simulink model "Position_MPC_Adaptive_OuterLoop"  (R2018a)
settings: Solver=VariableStepAuto  StartTime=0.0  StopTime=inf  FixedStep=0.01  RelTol=1e-3  EnableMultiTasking=on
PreLoadFcn:
  | sampleTime = 0.05;
  | 
  | % Vehicle Parameters
  | R = 0.1;
  | L = 0.5;
undefined symbols (not defined in the file): Ad, Bd, Beta, C1, C2, cBW, d, dw, Kb, Kg, Kt, La, mc, Ra, Waypoint
libraries: mobileRoboticsLib x2, mpclib x1, cstblocks x1, dspsrcs4 x1
settings Model: SimulationMode=accelerator  EnablePacing=on  Creator=scastro  LastModifiedBy=shravan
settings DataIOCC: LimitDataPoints=on
settings OptimizationCC: LifeSpan=inf
settings DebuggingCC: AllowSymbolicDim=off  SFUnexpectedBacktrackingDiag=warning  SFNoUnconditionalDefaultTransitionDiag=warning  SFExecutionAtInitializationDiag=none
settings CodeAppCC: StateflowObjectComments=on
settings GRTTargetCC: TargetLangStandard=C89/C90 (ANSI)  GeneratePreprocessorConditionals=Disable all
settings ConfigComp: CovMetricSettings=dw  CovHtmlReporting=on  CovSaveCumulativeToWorkspaceVar=on  CovSaveSingleToWorkspaceVar=on  CovExternalEMLEnable=off  CovSFcnEnable=off
settings SimscapeCC: SimscapeNominalValues="[{\"value\":\"10\",\"unit\":\"V\"},{\"value\":\"1\",\"unit\":\"A\"},{\"value\":\"10\",\"unit\":\"N*m\"},{\"value\":\"10\",\"unit\":\"bar\"},{\"value\":\"100\",\"unit\":\"kJ/kg\"},{\"value\":\"1\",\"unit\":\"kW\"},{\"value\":\"300\",\"unit\":\"K\"},{\"value\":\"100\",\"unit\":\"cm^3/s\"},{\"value\":\"1\",\"unit\":\"kN\"},{\"value\":\"1\",\"unit\":\"g/cm^3\"},{\"value\":\"1\",\"unit\":\"l\"},{\"value\":\"1\",\"unit\":\"cm^2\"},{\"value\":\"60\",\"unit\":\"Hz\"}]"  SimscapeLogType=all  SimscapeLogDataHistory=10000
settings ConfigurationSet: Description=SimMechanics 2G
settings ExplorerConfigSet: InternalSimMechanicsExplorerSettings="<ExplorerConfiguration><canonicalview>default</canonicalview><AnimationSetting><BasePlaybackSpeed>1.0</BasePlaybackSpeed><PlaybackSpeedFactor>1.0</PlaybackSpeedFactor></AnimationSetting><TilePanel><TileInfo><Tiles Columns=\"1\" Count=\"1\" Rows=\"1\"><Column Weight=\"1\"/><Row Weight=\"1\"/><Tile Height=\"1\" Width=\"1\" X=\"0\" Y=\"0\"/></Tiles></TileInfo><SceneInfo><SceneViewer><BGColor><R>0.60000002384185791</R><G>0.60000002384185791</G><B>0.60000002384185791</B></BGColor><Camera><DoPerspective>off</DoPerspective><Position><X>-1.70656042355848525</X><Y>-0.974920623359631922</Y><Z>4.72930454537082046</Z></Position><Center><X>0.552860638431633689</X><Y>1.42025063411503494</Y><Z>1.4843509506914252</Z></Center><Up><X>0.664249622453917166</X><Y>0.300615402055903091</Y><Z>0.684399604848363485</Z></Up><ViewLimDist>1</ViewLimDist><YLim>2.77881717169207398</YLim><XLim>3.55928742670435394</XLim></Camera></SceneViewer></SceneInfo></TilePanel><MechEditorPanel><Cameras/><GfxPanelCameraMap/><VideoCreator><PlaybackSpeedRatio>1.0</PlaybackSpeedRatio><FrameRate>30</FrameRate><VideoFormat>Motion JPEG AVI</VideoFormat><FrameSize>auto</FrameSize></VideoCreator></MechEditorPanel></ExplorerConfiguration>"

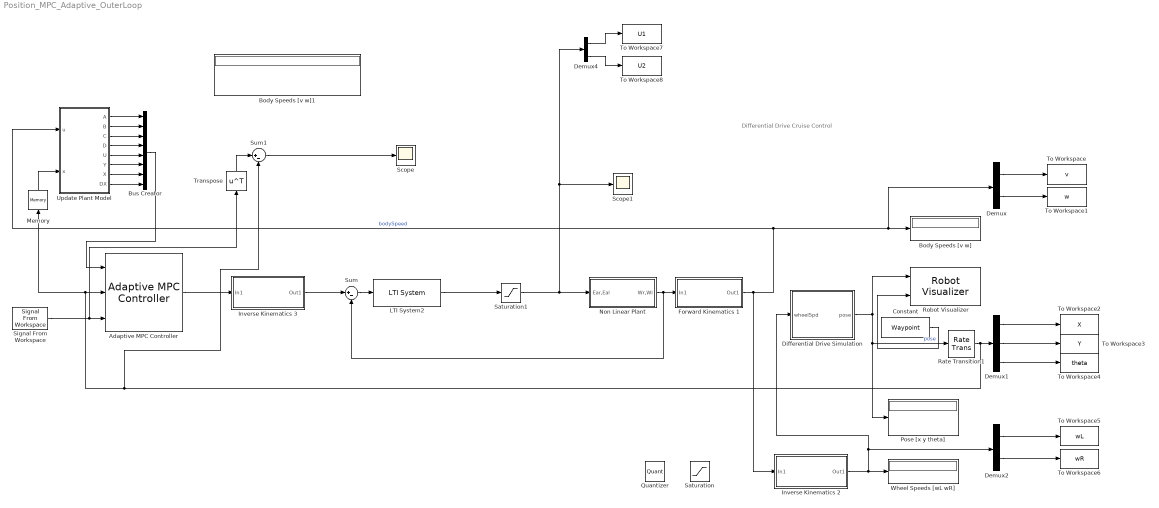
== system Position_MPC_Adaptive_OuterLoop ==
  note: Differential Drive Cruise Control
  Adaptive MPC Controller : mpclib/Adaptive MPC Controller  SCDEnableBlockLinearizationSpecification=on  mpcobj=mpc1  updateMPCinCallerWorkspace=on  md_inport=off  mv_inport=off  cost_outport=off  return_sequence=off  return_qpstatus=off  return_state=off  state_inport=off  isltv_plant=off  lims_inport=off  cc_inport=off  ywt_inport=off  uwt_inport=off  duwt_inport=off  rhoeps_inport=off  uref_inport=off  BlockDataType=double  SampleTimeInherited=off  switch_inport=off
      settings: SourceProductName=Model Predictive Control Toolbox
  Body Speeds [v w] : Display
  Body Speeds [v w]1 : Display
  Bus Creator : BusCreator  Inputs=8
  Constant : Constant  Value=Waypoint  SampleTime=sampleTime
  Demux : Demux  Outputs=2
  Demux1 : Demux  Outputs=3
  Demux2 : Demux  Outputs=2
  Demux4 : Demux  Outputs=2
  Differential Drive Simulation : Subsystem  AncestorBlock=mobileRoboticsLib/Kinematic Models/Differential Drive/Differential Drive Simulation  OverrideUsingVariant=mode==2  mask(Differential Drive Simulation){wheelRadius=R, wheelBase=dw, initX=C1, initY=C2, initAngle=0, Ts=0}
      mask prompts: wheelRadius "Wheel Radius [m]"; wheelBase "Wheelbase [m]"; initX "Initial X Position [m]"; initY "Initial Y Position [m]"; initAngle "Initial Angle [rad]"; Ts "Sample Time"
      mask help:
      | Simulates the kinematics of a differential drive vehicle from a specified initial pose.
      |
      | Input: Left and right wheel speeds [wL; wR], in rad/s
      |
      | Output: Pose [x; y; theta], in m, m, and rad
      |
      | Set the Sample Time parameter to 0 for continuous-time simulation, or a positive number for discrete-time simulation.
      mask Help: web('matlab:edit mrsDocDifferentialDrive')
      mask Callback Ts:
      | Ts = evalin('base',get_param(gcb,'Ts'));
      | blk = [gcb '/Generic Robot Simulation/Velocity Integrator'];
      | if Ts > 0
      |     set_param(blk,'OverrideUsingVariant','mode==2');
      | else
      |     set_param(blk,'OverrideUsingVariant','mode==1');
      | end
  Forward Kinematics 1 : Subsystem
  Inverse Kinematics 2 : Subsystem
  Inverse Kinematics 3 : Subsystem
  LTI System2 : cstblocks/LTI System  sys=Controller  IC=[]
  Memory : Memory
  "Non Linear Plant " : Subsystem
  Pose [x y theta] : Display
  Quantizer : Quantizer
  Rate Transition1 : RateTransition  OutPortSampleTime=0.01
  Robot Visualizer : mobileRoboticsLib/Environments/Robot Visualizer  Priority=99  robotRadius=1  showTrajectory=on  hasWaypoints=on  hasLidar=off  sensorOffset=[ 0 0 ]  scanAngles=[-pi/4,0,pi/4]  hasObjDetector=off  objDetectorOffset=[ 0, 0 ]  objDetectorAngle=0  objDetectorFOV=pi/4  objDetectorMaxRange=5  objectColors=[ 1, 0, 0; 0, 1, 0; 0, 0, 1 ]  objectMarkers='s'
      settings: SourceProductName=Mobile Robotics Simulation Library
  Saturation : Saturate
  Saturation1 : Saturate  UpperLimit=30  LowerLimit=-30
  Scope : Scope
  Scope1 : Scope
  Signal From Workspace : dspsrcs4/Signal From Workspace  X=Lyapunov  Ts=cBW  nsamps=1  OutputAfterFinalValue=Holding final value  ignoreOrWarnInputAndFrameLengths=off  OutputFrames=off
  Sum : Sum  Inputs=|+-
  Sum1 : Sum  Inputs=|+-
  To Workspace : ToWorkspace  VariableName=v  SampleTime=-1
  To Workspace1 : ToWorkspace  VariableName=w  SampleTime=-1
  To Workspace2 : ToWorkspace  VariableName=X  SampleTime=-1
  To Workspace3 : ToWorkspace  VariableName=Y  SampleTime=-1
  To Workspace4 : ToWorkspace  VariableName=theta  SampleTime=-1
  To Workspace5 : ToWorkspace  VariableName=wL  SampleTime=-1
  To Workspace6 : ToWorkspace  VariableName=wR  SampleTime=-1
  To Workspace7 : ToWorkspace  VariableName=U1  SaveFormat=Timeseries  SampleTime=-1
  To Workspace8 : ToWorkspace  VariableName=U2  SaveFormat=Timeseries  SampleTime=-1
  Transpose : Math  Operator=transpose  SaturateOnIntegerOverflow=on
  Update Plant Model : MATLAB Function  TreatAsAtomicUnit=on  SystemSampleTime=0.01
  Wheel Speeds [wL wR] : Display
  wires:
  Differential Drive Simulation/1(pose) -> Rate Transition1/1, Pose [x y theta]/1, Robot Visualizer/1  "pose"
  Forward Kinematics 1/1(Out1) -> Update Plant Model/1(u), Demux/1, Body Speeds [v w]/1, Inverse Kinematics 2/1(In1)  "bodySpeed"
  Demux/1 -> To Workspace/1
  Demux/2 -> To Workspace1/1
  Demux1/1 -> To Workspace2/1
  Demux1/2 -> To Workspace3/1
  Demux2/1 -> To Workspace5/1
  Demux2/2 -> To Workspace6/1
  Constant/1 -> Robot Visualizer/2
  Sum/1 -> LTI System2/1
  Demux1/3 -> To Workspace4/1
  Inverse Kinematics 2/1(Out1) -> Differential Drive Simulation/1(wheelSpd), Demux2/1, Wheel Speeds [wL wR]/1
  "Non Linear Plant "/1(Wr,Wl) -> Forward Kinematics 1/1(In1), Sum/2
  Rate Transition1/1 -> Sum1/2, Memory/1, Adaptive MPC Controller/2, Demux1/1
  Saturation1/1 -> "Non Linear Plant "/1(Ear,Eal), Scope1/1, Demux4/1
  Demux4/1 -> To Workspace7/1
  Demux4/2 -> To Workspace8/1
  Inverse Kinematics 3/1(Out1) -> Sum/1
  LTI System2/1 -> Saturation1/1
  Update Plant Model/1(A) -> Bus Creator/1
  Update Plant Model/2(B) -> Bus Creator/2
  Update Plant Model/3(C) -> Bus Creator/3
  Update Plant Model/4(D) -> Bus Creator/4
  Update Plant Model/5(U) -> Bus Creator/5
  Update Plant Model/6(Y) -> Bus Creator/6
  Update Plant Model/7(X) -> Bus Creator/7
  Update Plant Model/8(DX) -> Bus Creator/8
  Bus Creator/1 -> Adaptive MPC Controller/1
  Memory/1 -> Update Plant Model/2(x)
  Sum1/1 -> Scope/1
  Signal From Workspace/1 -> Transpose/1, Adaptive MPC Controller/3
  Transpose/1 -> Sum1/1
  Adaptive MPC Controller/1 -> Inverse Kinematics 3/1(In1)

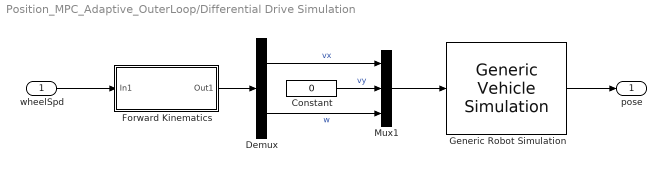
== system Position_MPC_Adaptive_OuterLoop/Differential Drive Simulation ==
  wheelSpd : Inport
  Constant : Constant  Value=0
  Demux : Demux  Outputs=2
  "Forward Kinematics " : Subsystem
  Generic Robot Simulation : mobileRoboticsLib/Utilities/Generic Vehicle Simulation  initX=initX  initY=initY  initAngle=initAngle  Ts=Ts
      link override Velocity Integrator: OverrideUsingVariant=mode==1
      settings: SourceProductName=Mobile Robotics Simulation Toolbox
  Mux1 : Mux  Inputs=3
  pose : Outport
  wires:
  Generic Robot Simulation/1 -> pose/1
  "Forward Kinematics "/1(Out1) -> Demux/1
  wheelSpd/1 -> "Forward Kinematics "/1(In1)
  Constant/1 -> Mux1/2  "vy"
  Demux/2 -> Mux1/3  "w"
  Demux/1 -> Mux1/1  "vx"
  Mux1/1 -> Generic Robot Simulation/1

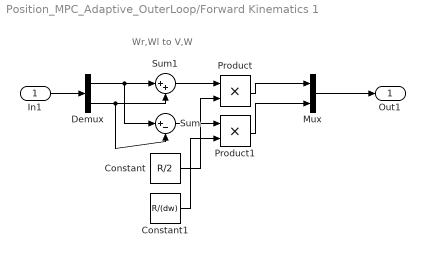
== system Position_MPC_Adaptive_OuterLoop/Forward Kinematics 1 ==
  note: Wr,Wl to V,W
  In1 : Inport
  Constant : Constant  Value=R/2
  Constant1 : Constant  Value=R/(dw)
  Demux : Demux  Outputs=2
  Mux : Mux  Inputs=2
  Product : Product
  Product1 : Product
  Sum : Sum  Inputs=|+-
  Sum1 : Sum  Inputs=|++
  Out1 : Outport
  wires:
  Constant1/1 -> Product1/2
  Sum/1 -> Product1/1
  Constant/1 -> Product/2
  Sum1/1 -> Product/1
  Demux/2 -> Sum1/2, Sum/2
  Demux/1 -> Sum1/1, Sum/1
  Product/1 -> Mux/1
  Mux/1 -> Out1/1
  Product1/1 -> Mux/2
  In1/1 -> Demux/1

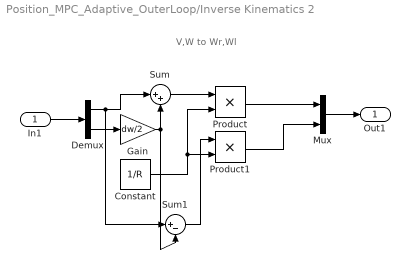
== system Position_MPC_Adaptive_OuterLoop/Inverse Kinematics 2 ==
  note: V,W to Wr,Wl
  In1 : Inport
  Constant : Constant  Value=1/R
  Demux : Demux  Outputs=2
  Gain : Gain  Gain=dw/2
  Mux : Mux  Inputs=2
  Product : Product
  Product1 : Product
  Sum : Sum  Inputs=|++
  Sum1 : Sum  Inputs=|+-
  Out1 : Outport
  wires:
  Gain/1 -> Sum/2, Sum1/2
  Product1/1 -> Mux/2
  Product/1 -> Mux/1
  Sum1/1 -> Product1/1
  Constant/1 -> Product/2, Product1/2
  Sum/1 -> Product/1
  Demux/1 -> Sum/1, Sum1/1
  Demux/2 -> Gain/1
  In1/1 -> Demux/1
  Mux/1 -> Out1/1

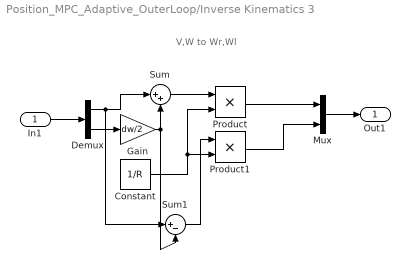
== system Position_MPC_Adaptive_OuterLoop/Inverse Kinematics 3 ==
  note: V,W to Wr,Wl
  In1 : Inport
  Constant : Constant  Value=1/R
  Demux : Demux  Outputs=2
  Gain : Gain  Gain=dw/2
  Mux : Mux  Inputs=2
  Product : Product
  Product1 : Product
  Sum : Sum  Inputs=|++
  Sum1 : Sum  Inputs=|+-
  Out1 : Outport
  wires:
  Gain/1 -> Sum/2, Sum1/2
  Product1/1 -> Mux/2
  Product/1 -> Mux/1
  Sum1/1 -> Product1/1
  Constant/1 -> Product/2, Product1/2
  Sum/1 -> Product/1
  Demux/1 -> Sum/1, Sum1/1
  Demux/2 -> Gain/1
  In1/1 -> Demux/1
  Mux/1 -> Out1/1

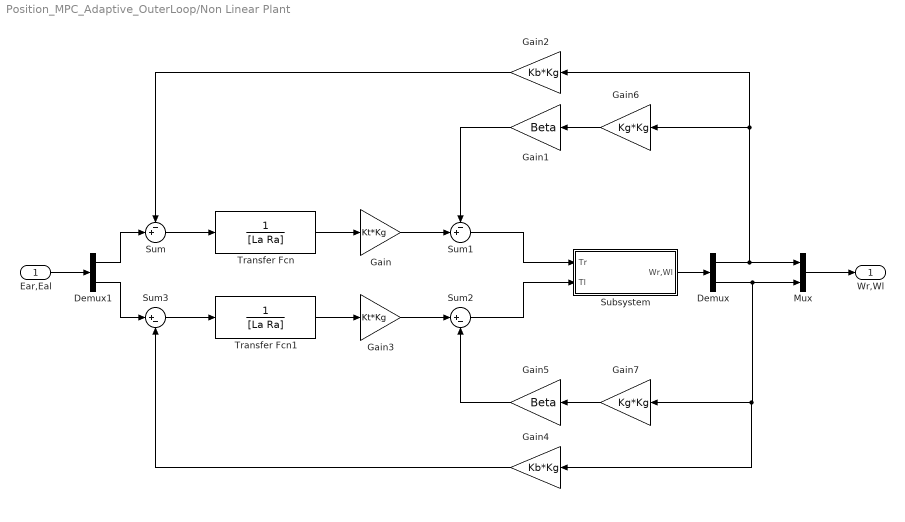
== system Position_MPC_Adaptive_OuterLoop/Non Linear Plant  ==
  Ear,Eal : Inport
  Demux : Demux  Outputs=2
  Demux1 : Demux  Outputs=2
  Gain : Gain  Gain=Kt*Kg
  Gain1 : Gain  Gain=Beta
  Gain2 : Gain  Gain=Kb*Kg
  Gain3 : Gain  Gain=Kt*Kg
  Gain4 : Gain  Gain=Kb*Kg
  Gain5 : Gain  Gain=Beta
  Gain6 : Gain  Gain=Kg*Kg
  Gain7 : Gain  Gain=Kg*Kg
  Mux : Mux  Inputs=2
  Subsystem : Subsystem
  Sum : Sum  Inputs=-+|
  Sum1 : Sum  Inputs=-+|
  Sum2 : Sum  Inputs=|+-
  Sum3 : Sum  Inputs=|+-
  Transfer Fcn : TransferFcn  Denominator=[La Ra]
  Transfer Fcn1 : TransferFcn  Denominator=[La Ra]
  Wr,Wl : Outport
  wires:
  Gain5/1 -> Sum2/2
  Gain4/1 -> Sum3/2
  Sum/1 -> Transfer Fcn/1
  Demux1/2 -> Sum3/1
  Gain1/1 -> Sum1/1
  Demux/1 -> Mux/1, Gain2/1, Gain6/1
  Subsystem/1(Wr,Wl) -> Demux/1
  Demux1/1 -> Sum/2
  Sum3/1 -> Transfer Fcn1/1
  Mux/1 -> Wr,Wl/1
  Gain2/1 -> Sum/1
  Gain/1 -> Sum1/2
  Ear,Eal/1 -> Demux1/1
  Sum1/1 -> Subsystem/1(Tr)
  Transfer Fcn/1 -> Gain/1
  Transfer Fcn1/1 -> Gain3/1
  Gain3/1 -> Sum2/1
  Demux/2 -> Mux/2, Gain4/1, Gain7/1
  Sum2/1 -> Subsystem/2(Tl)
  Gain6/1 -> Gain1/1
  Gain7/1 -> Gain5/1

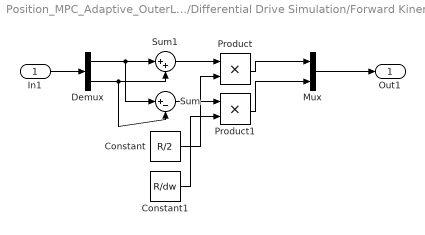
== system Position_MPC_Adaptive_OuterLoop/Differential Drive Simulation/Forward Kinematics  ==
  In1 : Inport
  Constant : Constant  Value=R/2
  Constant1 : Constant  Value=R/dw
  Demux : Demux  Outputs=2
  Mux : Mux  Inputs=2
  Product : Product
  Product1 : Product
  Sum : Sum  Inputs=|+-
  Sum1 : Sum  Inputs=|++
  Out1 : Outport
  wires:
  In1/1 -> Demux/1
  Product1/1 -> Mux/2
  Mux/1 -> Out1/1
  Product/1 -> Mux/1
  Demux/1 -> Sum/1, Sum1/1
  Demux/2 -> Sum/2, Sum1/2
  Sum1/1 -> Product/1
  Constant/1 -> Product/2
  Sum/1 -> Product1/1
  Constant1/1 -> Product1/2

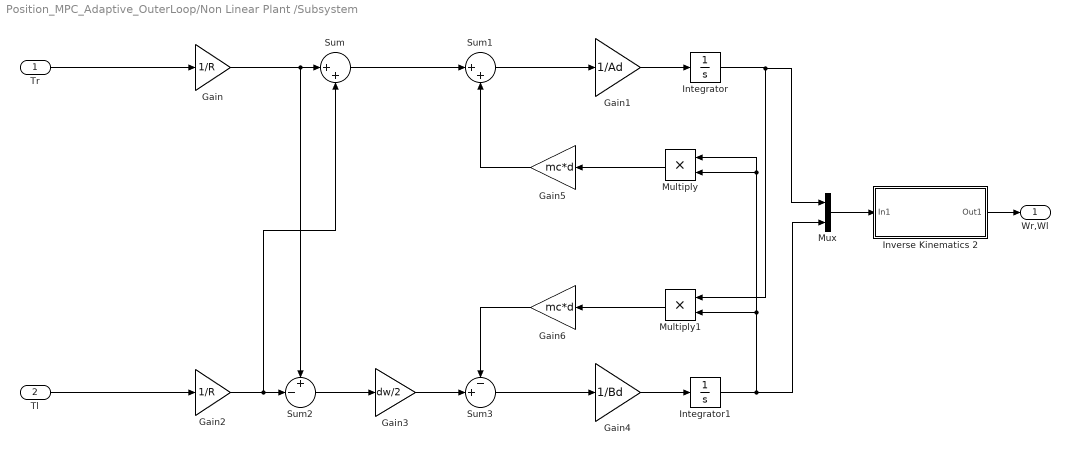
== system Position_MPC_Adaptive_OuterLoop/Non Linear Plant /Subsystem ==
  Tr : Inport
  Tl : Inport  Port=2
  Gain : Gain  Gain=1/R
  Gain1 : Gain  Gain=1/Ad
  Gain2 : Gain  Gain=1/R
  Gain3 : Gain  Gain=dw/2
  Gain4 : Gain  Gain=1/Bd
  Gain5 : Gain  Gain=mc*d
  Gain6 : Gain  Gain=mc*d
  Integrator : Integrator
  Integrator1 : Integrator
  Inverse Kinematics 2 : Subsystem
  Multiply : Product
  Multiply1 : Product
  Mux : Mux  Inputs=2
  Sum : Sum  Inputs=|++
  Sum1 : Sum  Inputs=|++
  Sum2 : Sum  Inputs=+-|
  Sum3 : Sum  Inputs=-+|
  Wr,Wl : Outport
  wires:
  Sum1/1 -> Gain1/1
  Multiply1/1 -> Gain6/1
  Sum3/1 -> Gain4/1
  Gain/1 -> Sum/1, Sum2/1
  Integrator/1 -> Mux/1, Multiply1/1
  Mux/1 -> Inverse Kinematics 2/1(In1)
  Gain4/1 -> Integrator1/1
  Inverse Kinematics 2/1(Out1) -> Wr,Wl/1
  Sum/1 -> Sum1/1
  Gain5/1 -> Sum1/2
  Tr/1 -> Gain/1
  Integrator1/1 -> Multiply1/2, Multiply/2, Multiply/1, Mux/2
  Multiply/1 -> Gain5/1
  Gain3/1 -> Sum3/2
  Sum2/1 -> Gain3/1
  Gain2/1 -> Sum/2, Sum2/2
  Gain6/1 -> Sum3/1
  Tl/1 -> Gain2/1
  Gain1/1 -> Integrator/1

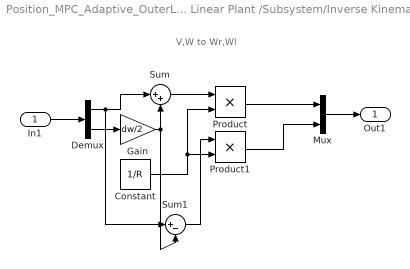
== system Position_MPC_Adaptive_OuterLoop/Non Linear Plant /Subsystem/Inverse Kinematics 2 ==
  note: V,W to Wr,Wl
  In1 : Inport
  Constant : Constant  Value=1/R
  Demux : Demux  Outputs=2
  Gain : Gain  Gain=dw/2
  Mux : Mux  Inputs=2
  Product : Product
  Product1 : Product
  Sum : Sum  Inputs=|++
  Sum1 : Sum  Inputs=|+-
  Out1 : Outport
  wires:
  Mux/1 -> Out1/1
  In1/1 -> Demux/1
  Demux/2 -> Gain/1
  Demux/1 -> Sum1/1, Sum/1
  Gain/1 -> Sum1/2, Sum/2
  Sum/1 -> Product/1
  Constant/1 -> Product1/2, Product/2
  Sum1/1 -> Product1/1
  Product/1 -> Mux/1
  Product1/1 -> Mux/2

== matlab function Position_MPC_Adaptive_OuterLoop/Update Plant Model ==
  data: u input size=[2,1]; A output size=[3,3]; x input size=[3,1]; B output size=[3,2]; C output size=[3,3]; D output size=[3,2]; U output size=[2,1]; Y output size=[3,1]; X output size=[3,1]; DX output size=[3,1]
function [A,B,C,D,U,Y,X,DX] = fcn(u,x)
% Sample time
Ts = 0.01;

% Model parameters
U1eq = u(1);
Thetaeq = x(3);

% Continuous-time model
Ac = [0 0 0;
      0 0 0;
      0 0 0];
Bc = [cos(Thetaeq) 0;
      sin(Thetaeq) 0;
      0            1];   
Cc = [1 0 0; 0 1 0; 0 0 1];
Dc = zeros(3,2);

% Generate discrete-time model
nx = size(Ac,1);
nu = size(Bc,2);
M = expm([[Ac Bc]*Ts; zeros(nu,nx+nu)]);
A = M(1:nx,1:nx);
B = M(1:nx,nx+1:nx+nu);
C = Cc;
D = Dc;

% Nominal conditions for discrete-time plant
X = x;
U = u;
Y = C*x + D*u;
DX = A*x+B*u-x;
